simulink model "ST5B_Informativity"  (R2020a)
settings: Solver=ode8  StartTime=0.0  StopTime=4.5  FixedStep=0.005  RelTol=1e-3
values from neighbouring files (symbols this model uses):
  Efd0 = 1.3468515    [AVR.m]    (also in AVR_parameter_change.m = Efd(1))
  Kc = 0.95    [AVR.m]    (also in AVR_parameter_change.m = 1)
  Kr = 500    [AVR.m]    (also in AVR_parameter_change.m)
  T1 = 0.005    [AVR.m]    (also in AVR_parameter_change.m)
  Tr = 0.01    [AVR.m]    (also in AVR_parameter_change.m)
  V = V(1:901)    [AVR.m]    (also in AVR_parameter_change.m = V-mean(V(1:10)); PSS_ON.mat = [0.987464272 0.987408927 0.987298238 0.987574962 0.987464272; PSS_ON_Dymola.mat = [0.987464272 0.987408927 0.987298238 0.987574962 0.987464272; PSS_ON_short.mat = [0 1.4652769e-10 5.5672267e-10 1.1685104e-09 1.9773894e-09 2)
  Vinit = V(1)    [AVR.m]    (also in AVR_parameter_change.m)
  VR0 = Efd0 + Kc*XadIfd    [AVR.m]    (also in AVR_parameter_change.m)
  Vrmax = 4.35    [AVR.m]    (also in AVR_parameter_change.m)
  Vrmin = -3.825    [AVR.m]    (also in AVR_parameter_change.m)
  XadIfd = Ifd(1)    [AVR.m]    (also in AVR_parameter_change.m; Xd_13013.mat = ; generator.m = Xad*Ifd)
libraries: eeGeneralControl x4, simulink x1
settings Model: Creator=meagh  LastModifiedBy=meagh

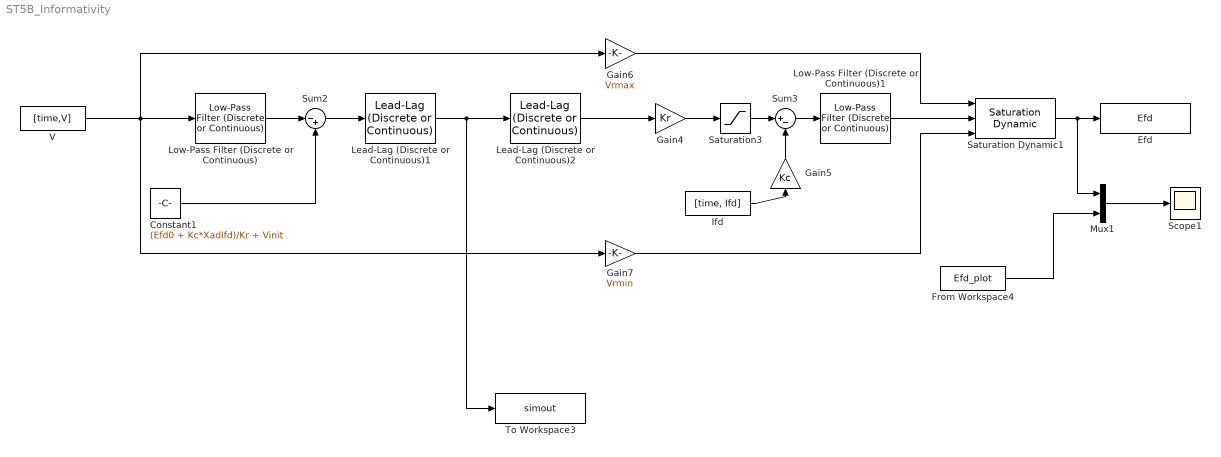
== system ST5B_Informativity ==
  Constant1 : Constant  Value=(Efd0 + Kc*XadIfd)/Kr + Vinit
  Efd : ToWorkspace  VariableName=Efd  SaveFormat=Timeseries  SampleTime=-1
  From Workspace4 : FromWorkspace  VariableName=Efd_plot
  Gain4 : Gain  Gain=Kr
  Gain5 : Gain  Gain=Kc
  Gain6 : Gain  Gain=Vrmax
  Gain7 : Gain  Gain=Vrmin
  Ifd : FromWorkspace  VariableName=[time, Ifd]
  Lead-Lag (Discrete or Continuous)1 : eeGeneralControl/Lead-Lag (Discrete or Continuous)  T1=Tc1  T2=Tb1  B=Vrmax/Kr  A=Vrmin/Kr  init_option=Specify as parameter  x0=VR0/Kr  Ts=-1
      settings: SourceProductBaseCode=PS
  Lead-Lag (Discrete or Continuous)2 : eeGeneralControl/Lead-Lag (Discrete or Continuous)  T1=Tc2  T2=Tb2  B=Vrmax/Kr  A=Vrmin/Kr  init_option=Specify as parameter  x0=VR0/Kr  Ts=-1
      settings: SourceProductBaseCode=PS
  Low-Pass Filter (Discrete or Continuous) : eeGeneralControl/Low-Pass Filter (Discrete or Continuous)  K=1  T=Tr  B=inf  A=-inf  init_option=Specify as parameter  x0=V(1)  Ts=0
  Low-Pass Filter (Discrete or Continuous)1 : eeGeneralControl/Low-Pass Filter (Discrete or Continuous)  K=1  T=T1  B=inf  A=-inf  init_option=Inherited from block input  x0=Efd0  Ts=-1
  Mux1 : Mux  Inputs=2
  Saturation Dynamic1 : simulink/Discontinuities/Saturation Dynamic  OutMin=[]  OutMax=[]  OutDataTypeStr=Inherit: Same as second input  OutDataType=fixdt(1, 16)  OutScaling=2^-10  DoSatur=off
  Saturation3 : Saturate  UpperLimit=Vrmax  LowerLimit=Vrmin  LinearizeAsGain=off
  Scope1 : Scope
  Sum2 : Sum  Inputs=|-+
  Sum3 : Sum  Inputs=|+-
  To Workspace3 : ToWorkspace  VariableName=simout  SaveFormat=Timeseries  SampleTime=-1
  V : FromWorkspace  VariableName=[time,V]
  wires:
  Constant1/1 -> Sum2/2
  Ifd/1 -> Gain5/1
  Gain7/1 -> Saturation Dynamic1/3
  From Workspace4/1 -> Mux1/2
  Mux1/1 -> Scope1/1
  Saturation Dynamic1/1 -> Mux1/1, Efd/1
  Sum3/1 -> Low-Pass Filter (Discrete or Continuous)1/1
  Gain6/1 -> Saturation Dynamic1/1
  Saturation3/1 -> Sum3/1
  Gain5/1 -> Sum3/2
  V/1 -> Low-Pass Filter (Discrete or Continuous)/1, Gain7/1, Gain6/1
  Sum2/1 -> Lead-Lag (Discrete or Continuous)1/1
  Low-Pass Filter (Discrete or Continuous)/1 -> Sum2/1
  Low-Pass Filter (Discrete or Continuous)1/1 -> Saturation Dynamic1/2
  Gain4/1 -> Saturation3/1
  Lead-Lag (Discrete or Continuous)1/1 -> To Workspace3/1, Lead-Lag (Discrete or Continuous)2/1
  Lead-Lag (Discrete or Continuous)2/1 -> Gain4/1
